simulink model "task1"  (R2024a)
settings: Solver=VariableStepAuto  StartTime=0.0  StopTime=10.0  RelTol=1e-6
values from neighbouring files (symbols this model uses):
  A = [8, 1, 11; 4, 0, 4; -4, -3, -7]    [main.m]
  B = [-1; -3; 3]    [main.m]
  K = find_controller(A, B, sigma)    [main.m]
settings Model: Creator=alexivanov  LastModifiedBy=alexivanov

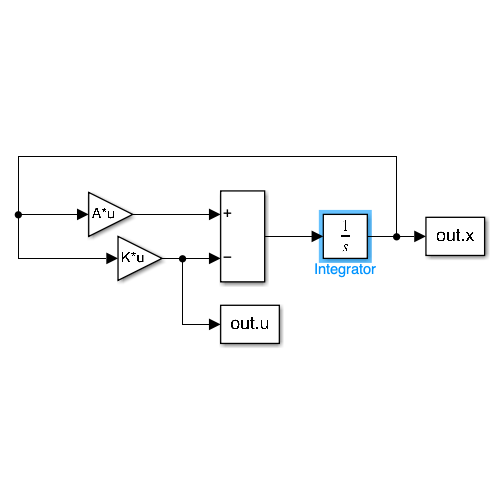
[thumbnail: Simulink's stored preview of the top-level diagram]
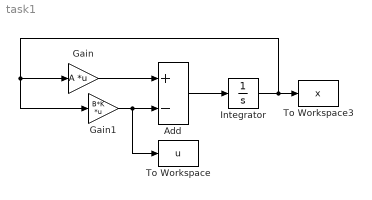
== system task1 ==
  Add : Sum  Inputs=+-
  Gain : Gain  Gain=A  Multiplication=Matrix(K*u)
  Gain1 : Gain  Gain=B*K  Multiplication=Matrix(K*u)
  Integrator : Integrator  InitialCondition=[1; 1; 1]
  To Workspace : ToWorkspace  VariableName=u  SampleTime=-1
  To Workspace3 : ToWorkspace  VariableName=x  SampleTime=-1
  wires:
  Integrator/1 -> Gain1/1, Gain/1, To Workspace3/1
  Gain/1 -> Add/1
  Gain1/1 -> To Workspace/1, Add/2
  Add/1 -> Integrator/1
